simulink library "RefChMixerBtc"  (R2022b)
settings: Solver=VariableStepAuto  StartTime=0.0  StopTime=10.0  RelTol=1e-3
libraries: TuneVar x3, FeaturePath x1, HandyTextFile x1
settings Model: Creator=kl13806  LastModifiedBy=kl13806
settings SolverCC: AlgebraicLoopSolver=TrustRegion
settings DebuggingCC: UnconnectedInputMsg=warning  UnconnectedOutputMsg=warning  UnconnectedLineMsg=warning  SFMachineParentedDataDiag=warning
settings ModelReferenceCC: EnableRefExpFcnMdlSchedulingChecks=on
settings RTWCC: DLArmComputeVersion=19.05

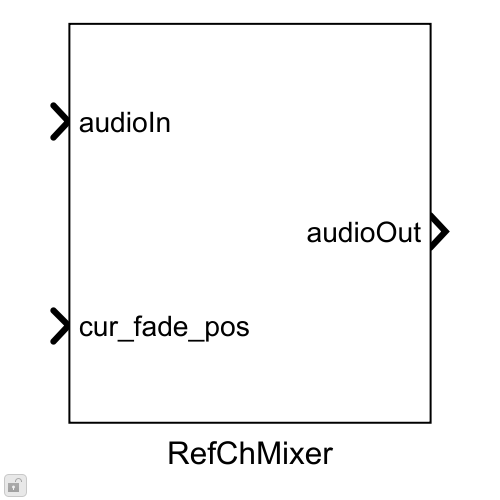
[thumbnail: Simulink's stored preview of the top-level diagram]
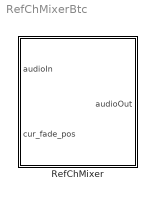
== system RefChMixerBtc ==
  RefChMixer : Subsystem  mask(Blocklib RefChMixer){Config=[], FeatureName=refChMixer}
      mask prompts: Config "RefChMixerConfig"; FeatureName "Feature path name:"
      mask help: Include fader flag is to select whether fader function is to be added or not for generating reference output
      mask init:
      | blkh=gcbh;
      | Config=BTConfig.Assert(blkh,Config);
      | 
      | Config.Validate();
      | BTConfig.InitSetFeatureIfPresent(blkh,'FeatureName');
      mask Callback Config: BTConfig.CallbackHideIfPresent(gcbh,{'FeatureName'});
      mask TypeOptions FeatureName: FeaturePath/FeatureName

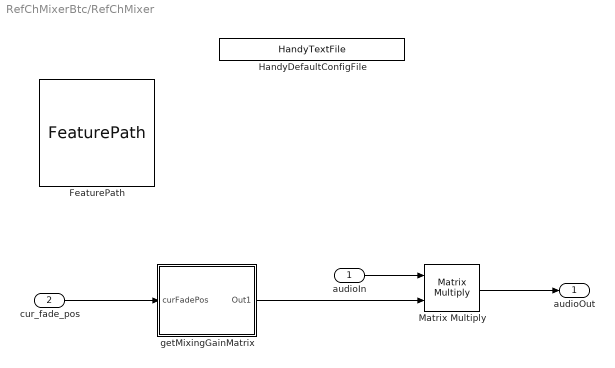
== system RefChMixerBtc/RefChMixer ==
  audioIn : Inport
  cur_fade_pos : Inport  Port=2
  FeaturePath : FeaturePath/FeaturePath  FeatureName=refChMixer  IsGroup=off  GroupNumber=-1  IsModule=off  TriggerInit=[-125 29 -10 136]
      settings: SourceProductName=Bose Talaria
  HandyDefaultConfigFile : HandyTextFile/HandyTextFile  TemplateSource=Config  FileSuffix=Init  OpenDialogOnLoad=off  UseThisBlockName=off  AddGrandParentNamePrefix=off  TheDefaultText=|  ShowInLibBrowser=on
      | % $(FILENAME) Setup model parameters for each "Init" callback (e.g. update diagram)
      | sample_rate_in_hertz = 44100;
      | frame_size = 32;
      | sysin_channel_count = 2;
      settings: SourceProductName=Bose Talaria
  Matrix Multiply : Product  Multiplication=Matrix(*)
  getMixingGainMatrix : Subsystem
  audioOut : Outport
  wires:
  getMixingGainMatrix/1(Out1) -> Matrix Multiply/2
  audioIn/1 -> Matrix Multiply/1
  Matrix Multiply/1 -> audioOut/1
  cur_fade_pos/1 -> getMixingGainMatrix/1(curFadePos)

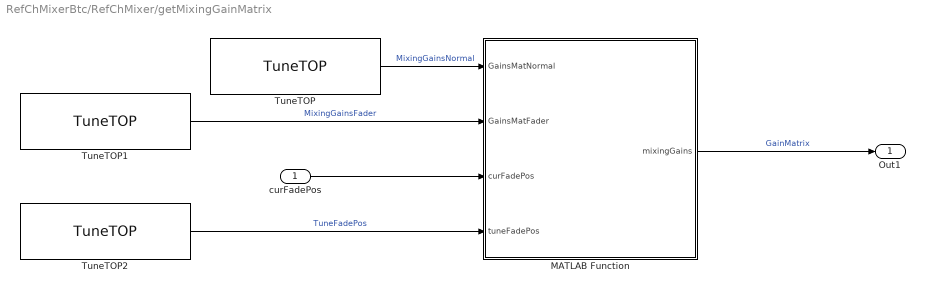
== system RefChMixerBtc/RefChMixer/getMixingGainMatrix ==
  curFadePos : Inport
  MATLAB Function : MATLAB Function  TreatAsAtomicUnit=on
  TuneTOP : TuneVar/TuneTOP  TriggerInit=[170 -63 340 -7]  TopName=MixingGainsNormal  TuneName=MixingGainsNormal  DataType=single  TunabilityNumber=1  MinValue=[]  MaxValue=[]  BankNumber=0  PreOverlay=false  PostOverlay=false  UseSameName=on  MaskValue=Config.DefaultMixingGainsNormal
      settings: SourceProductName=Bose Talaria
  TuneTOP1 : TuneVar/TuneTOP  TriggerInit=[-20 -8 150 48]  TopName=MixingGainsFader  TuneName=MixingGainsFader  DataType=single  TunabilityNumber=1  MinValue=[]  MaxValue=[]  BankNumber=0  PreOverlay=false  PostOverlay=false  UseSameName=on  MaskValue=Config.DefaultMixingGainsFader
      settings: SourceProductName=Bose Talaria
  TuneTOP2 : TuneVar/TuneTOP  TriggerInit=[-20 102 150 158]  TopName=TuneFadePos  TuneName=TuneFadePos  DataType=uint32  TunabilityNumber=1  MinValue=[]  MaxValue=[]  BankNumber=0  PreOverlay=false  PostOverlay=false  UseSameName=on  MaskValue=Config.DefaultTuneFadePos
      settings: SourceProductName=Bose Talaria
  Out1 : Outport
  wires:
  TuneTOP1/1 -> MATLAB Function/2(GainsMatFader)  "MixingGainsFader"
  MATLAB Function/1(mixingGains) -> Out1/1  "GainMatrix"
  TuneTOP/1 -> MATLAB Function/1(GainsMatNormal)  "MixingGainsNormal"
  curFadePos/1 -> MATLAB Function/3(curFadePos)
  TuneTOP2/1 -> MATLAB Function/4(tuneFadePos)  "TuneFadePos"

== matlab function RefChMixerBtc/RefChMixer/getMixingGainMatrix/MATLAB Function ==
  data: GainsMatNormal input; mixingGains output; GainsMatFader input; curFadePos input; includeFade parameter; tuneFadePos input
function mixingGains  = fcn(GainsMatNormal,GainsMatFader, curFadePos, includeFade, tuneFadePos)
%#codegen
% Check if includeFade is enabled
if(includeFade)
  % If enables assign the value to mixingGains based on the tuneFadePos
  if(curFadePos <= tuneFadePos)         
      mixingGains = GainsMatNormal';       
  else
      mixingGains = GainsMatFader';
  end  
else
  mixingGains = GainsMatNormal';
end
